simulink model "mtuner_control"  (Simulink 3.00)
settings: Solver=ode45  StartTime=0.0  StopTime=10.0  RelTol=1e-3
libraries: mathlib x7, genlib x5, execlib x3, reglib x3, analoglib x1, arclib x1
settings Model: LastModifiedBy=mertlj

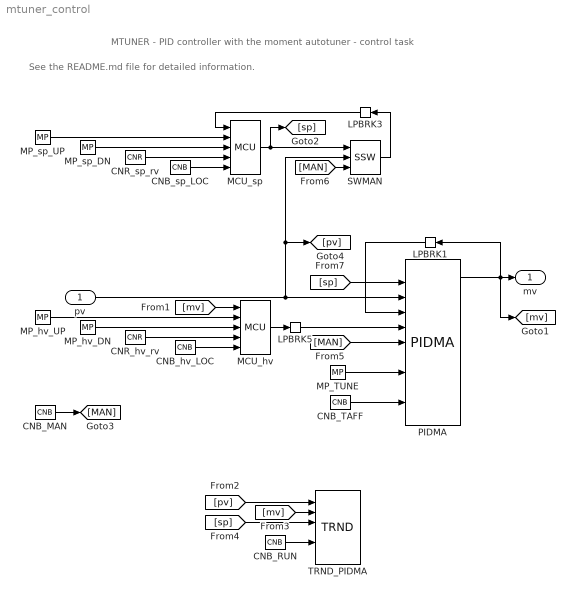
== system mtuner_control ==
  note: See the README.md file for detailed information.
  note: MTUNER - PID controller with the moment autotuner - control task
  pv : Inport  Port=1
  CNB_MAN : mathlib/CNB  YCN=off
  CNB_RUN : mathlib/CNB  YCN=on
  CNB_TAFF : mathlib/CNB  YCN=on
  CNB_hv_LOC : mathlib/CNB  YCN=on
  CNB_sp_LOC : mathlib/CNB  YCN=on
  CNR_hv_rv : mathlib/CNR  ycn=0
  CNR_sp_rv : mathlib/CNR  ycn=0
  LPBRK1 : execlib/LPBRK  Orientation=left
  LPBRK3 : execlib/LPBRK  Orientation=left
  LPBRK5 : execlib/LPBRK
  MCU_hv : reglib/MCU  tt=1  tm=50  y0=0  q=5  ta=2  tf=8  SATF=off  hilim=100  lolim=-100
  MCU_sp : reglib/MCU  tt=1  tm=50  y0=0  q=5  ta=2  tf=8  SATF=off  hilim=100  lolim=-100
  MP_TUNE : genlib/MP  pwidth=0.1  BSTATE=off  RPTF=off
  MP_hv_DN : genlib/MP  pwidth=0.1  BSTATE=off  RPTF=off
  MP_hv_UP : genlib/MP  pwidth=0.1  BSTATE=off  RPTF=off
  MP_sp_DN : genlib/MP  pwidth=0.1  BSTATE=off  RPTF=off
  MP_sp_UP : genlib/MP  pwidth=0.1  BSTATE=off  RPTF=off
  PIDMA : reglib/PIDMA  co=AUTOTUNER  irtype=7: PID  RACT=off  k=1  ti=4  td=1  nd=10  b=1  c=0  tt=1  hilim=100  lolim=-100  dz=0  icotype=1: Analog  ittype=7: PID  iainf=1: Static process  DGC=on  tdg=10  tn=2  amp=10  dy=5  ispeed=1: Slow closed loop  ipid=1: Parallel form
  SWMAN : analoglib/SSW
  TRND_PIDMA : arclib/TRND  n=3  l=1000  btype=8: Double  ptype1=1: Store  ptype2=1: Store  ptype3=1: Store  ptype4=1: Store  pfac=1  afac=0  arc=0  id=1  Title=Trend Title  timesrc=1
  mv : Outport  Port=1
  wires:
  CNB_MAN/1 -> [MAN]
  CNB_RUN/1 -> TRND_PIDMA/5
  CNB_TAFF/1 -> PIDMA/10
  CNB_hv_LOC/1 -> MCU_hv/5
  CNB_sp_LOC/1 -> MCU_sp/5
  CNR_hv_rv/1 -> MCU_hv/4
  CNR_sp_rv/1 -> MCU_sp/4
  [mv] -> MCU_hv/1
  [pv] -> TRND_PIDMA/1
  [mv] -> TRND_PIDMA/2
  [sp] -> TRND_PIDMA/3
  [MAN] -> PIDMA/6
  [MAN] -> SWMAN/3
  [sp] -> PIDMA/2
  LPBRK1/1 -> PIDMA/4
  LPBRK3/1 -> MCU_sp/1
  LPBRK5/1 -> PIDMA/5
  MCU_hv/1 -> LPBRK5/1
  MCU_sp/1 -> [sp], SWMAN/1
  MP_TUNE/1 -> PIDMA/8
  MP_hv_DN/1 -> MCU_hv/3
  MP_hv_UP/1 -> MCU_hv/2
  MP_sp_DN/1 -> MCU_sp/3
  MP_sp_UP/1 -> MCU_sp/2
  PIDMA/1 -> [mv], LPBRK1/1, mv/1
  SWMAN/1 -> LPBRK3/1
  pv/1 -> PIDMA/3, [pv], SWMAN/2
